simulink model "DC_Microgrid_Sim"  (R2023b)
settings: Solver=VariableStepDiscrete  StartTime=0.0  StopTime=720  MaxStep=1e2  RelTol=1e-3
undefined symbols (not defined in the file or in its folder): Ion, Lithium, Ts_Control, Ts_Power
libraries: spsSeriesRLCBranchLib x5, spsVoltageMeasurementLib x3, spsCurrentMeasurementLib x2, spsMosfetLib x2, SignalEditorBlockLib x2, spsDiodeLib x2, spsFirstOrderFilterLib x2, spsBatteryLib x1, simulink x1, slpidlib x1, spsPWMGeneratorDCDCLib x1, spsVariableResistorLib x1
settings Model: SimulationMode=accelerator  Creator=andrewboland  LastModifiedBy=andrewboland

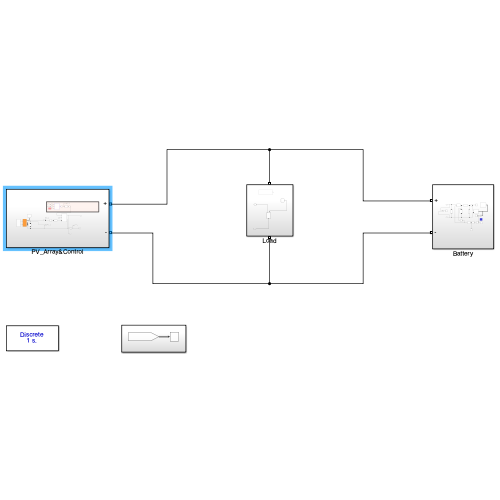
[thumbnail: Simulink's stored preview of the top-level diagram]
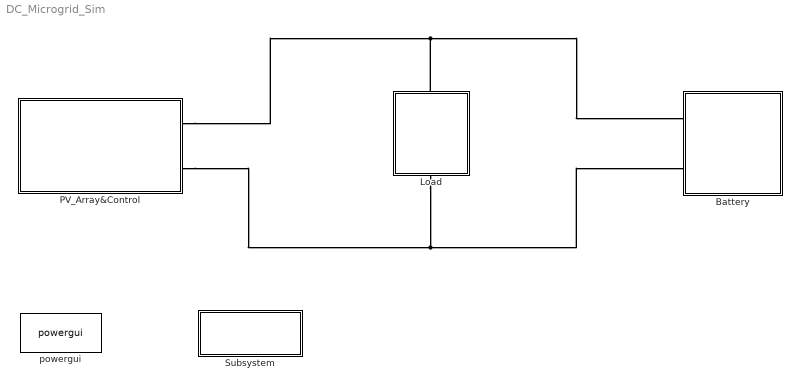
== system DC_Microgrid_Sim ==
  Battery : Subsystem
  Load : Subsystem
      settings: PortSchema="{\"entries\":[{\"content\":{\"sides\":[{\"content\":{},\"type\":\"ConnectorPlacement.EquallySpacedRectSide\",\"uuid\":\"223a8ec7-d9ac-4869-be30-0e3f111284b6\"},{\"content\":{\"side\":\"RIGHT\"},\"type\":\"ConnectorPlacement.EquallySpacedRectSide\",\"uuid\":\"4171ceb5-df16-4550-9af5-4849cdd8fb69\"},{\"content\":{\"connectorIds\":[\"LConn1\"],\"side\":\"TOP\"},\"type\":\"ConnectorPlacement.EquallySpacedRectSide\",\"uuid\":\"6a035cfa-8de8-4480-8689-7e250be4b844\"},{\"content\":{\"connectorIds\":[\"RConn1\"],\"side\":\"BOTTOM\"},\"type\":\"ConnectorPlacement.EquallySpacedRectSide\",\"uuid\":\"833ff93c-2ddd-4d5a-b476-72d44fccdab2\"}]},\"type\":\"ConnectorPlacement.EquallySpacedConnector\",\"uuid\":\"7d183c8c-61a7-4d89-b167-90b7ffe5dbe5\"}],\"packageUris\":[\"http://schema.mathworks.com/mf0/Connector/R2020b\"],\"version\":\"1.0\"}"
  PV_Array&Control : Subsystem
  Subsystem : Subsystem
  powergui : spspowerguiLib/powergui  Priority=1  SimulationMode=Discrete  SampleTime=1  frequency=60  Iterations=50  frequencyindice=0  Pbase=100e6  ErrMax=1e-4  UnitsV=kV  UnitsW=MW  buscounter=0  FunctionMessages=off  echomessages=off  EnableUseOfTLC=off  CurrentSourceSwitches=off  DisableSnubberDevices=off  DisableRonSwitches=off  DisableVfSwitches=off  DisplayEquations=off  AutomaticDiscreteSolvers=off  SolverType=Tustin/Backward Euler (TBE)  Interpol=off  ExternalGateDelay=off  methode=off  Ts=100  x0status=blocks  SPID=on  SwTol=0  HookPort=off  NonlinearTolerance=1e-4  nMaxIteration=100  ContinueOnMaxIteration=off  RestoreLinks=warning  ResistiveCurrentMeasurement=off  Frange=[0:2:500]  Ylog=off  Xlog=on  ShowGrid=off  save=off  variable=ZData  structure=0  ZoomFFT=off  StartTime=0.0  cycles=1  DisplayStyle=1  fundamental=60  FreqAxis=off  MaxFrequency=1000  frequencyindicesteady=1  RmsSteady=1  display=off
  connections:
  PV_Array&Control/RConn1 -- Load/LConn1 -- Battery/LConn1
  PV_Array&Control/RConn2 -- Load/RConn1 -- Battery/LConn2

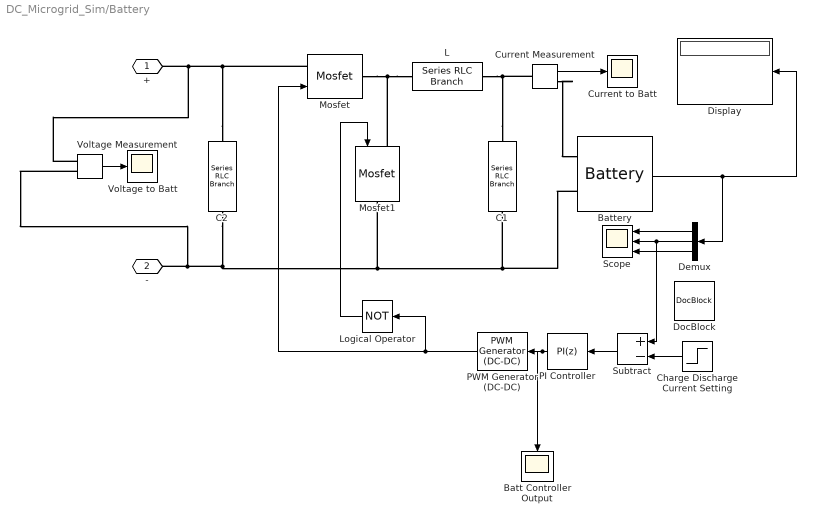
== system DC_Microgrid_Sim/Battery ==
  Batt Controller Output : Scope
  Battery : spsBatteryLib/Battery  BatType=Lithium-Ion  ShowTempParam=off  ThermalPreset=no  ShowAgeParam=off  NomV=400  NomQ=360  SOC=50  Batt_Tr=1  PresetModel=on  MaxQ=360  MinV=300  FullV=465.5949  Dis_rate=156.5217  R=0.011111  Normal_OP=325.5652  expZone="[432.1543      17.68696]"  current=[6.5 13 32.5]  Units=Time  Tci=20  NomT=25  T2=0  MaxQ2=2.208  FullV2=3.45  Normal_OP2=2.8  expZone2="[3.22        0.23]"  Rca=0.6  ti=1000  Dp=0  Neq0=0  Tsim=1e6  Ta1=25  Qeol=5.4*0.9  Reol=0.013333*1.2  Char_age=[2.3478, 3]  Dis_age=[2.3478, 10]  N1=1500  N2=10500  N3=1000  N4=1400  Ta2=45  N5=950
      settings: LibrarySourceBlock=electricdrivelib/Extra Sources/Battery
  C1 : spsSeriesRLCBranchLib/Series RLC Branch  LConnTagsString=__new0  RConnTagsString=__new0  BranchType=RC  Resistance=1e-3  Inductance=1e-3  SetiL0=off  InitialCurrent=0  Capacitance=1000e-6  Setx0=off  InitialVoltage=0  Measurements=None
  C2 : spsSeriesRLCBranchLib/Series RLC Branch  LConnTagsString=__new0  RConnTagsString=__new0  BranchType=RC  Resistance=1e-3  Inductance=1e-3  SetiL0=off  InitialCurrent=0  Capacitance=1000e-6  Setx0=off  InitialVoltage=0  Measurements=None
  Charge Discharge Current Setting : Step  Before=5  After=-5  SampleTime=0
  Current Measurement : spsCurrentMeasurementLib/Current Measurement  PhasorSimulation=off  OutputType=Complex  PSBequivalent=0
  Current to Batt : Scope
  Demux : Demux  Outputs=3
  Display : Display
  DocBlock : simulink/Model-Wide Utilities/DocBlock  DocumentType=Text
      content=|
      | Half Bridge Bidirectional DC-DC Converter with PI Current Control Demo
      | Developed by Rodney Tan (PhD)
      | Version 1.00 (July 2019)
      |
      | This Simulink model demonstrate a non-isolated half bridge Bidirectional
      | DC-DC Converter with PI current control typically used for battery charge
      | discharge control application.
      |
      | The charge and discharge mode is control by the charge discharge current
      | setting block where a positive current set the converter to discharging mode
      | and a negative current set the converter to charging mode.
  L : spsSeriesRLCBranchLib/Series RLC Branch  LConnTagsString=__new0  RConnTagsString=__new0  BranchType=L  Resistance=0.1  Inductance=100e-6  SetiL0=off  InitialCurrent=0  Capacitance=1e-6  Setx0=off  InitialVoltage=0  Measurements=None
  Logical Operator : Logic  Operator=NOT  AllPortsSameDT=off  OutDataTypeStr=boolean
  Mosfet : spsMosfetLib/Mosfet  Ron=0.1  Lon=0  Rd=0.01  Vfd=0  IC=0  Rs=1e5  Cs=inf  Measurements=off
  Mosfet1 : spsMosfetLib/Mosfet  Ron=0.1  Lon=0  Rd=0.01  Vfd=0  IC=0  Rs=1e5  Cs=inf  Measurements=off
  PI Controller : slpidlib/PID Controller  Controller=PI  Form=Parallel  TimeDomain=Discrete-time  UseExternalTs=off  SampleTime=-1  IntegratorMethod=Forward Euler  FilterMethod=Forward Euler  ControllerParametersSource=internal  P=0.01  I=5  UseKiTs=off  D=0  N=0  UseFilter=on  TunerSelectOption=Transfer Function Based (PID Tuner App)  InitialConditionSource=internal  InitialConditionForIntegrator=0  InitialConditionForFilter=0  DifferentiatorICPrevScaledInput=0  ExternalReset=none  TrackingMode=off  Kt=1  LimitOutput=on  SatLimitsSource=internal  UpperSaturationLimit=0.9  LowerSaturationLimit=0  LinearizeAsGain=on  AntiWindupMode=none  Kb=1  LimitIntegrator=off  UpperIntegratorSaturationLimit=inf  LowerIntegratorSaturationLimit=-inf  POutMin=[]  POutMax=[]  IOutMin=[]  IOutMax=[]  DOutMin=[]  DOutMax=[]  NOutMin=[]  NOutMax=[]  SumOutMin=[]  SumOutMax=[]  SaturationOutMin=[]  SaturationOutMax=[]  PParamMin=[]  PParamMax=[]  IParamMin=[]  IParamMax=[]  DParamMin=[]  DParamMax=[]  NParamMin=[]  NParamMax=[]  KbParamMin=[]  KbParamMax=[]  KtParamMin=[]  KtParamMax=[]  KbOutMin=[]  KbOutMax=[]  KtOutMin=[]  KtOutMax=[]  IntegratorOutMin=[]  IntegratorOutMax=[]  FilterOutMin=[]  FilterOutMax=[]  SumI1OutMin=[]  SumI1OutMax=[]  SumI2OutMin=[]  SumI2OutMax=[]  SumI3OutMin=[]  SumI3OutMax=[]  SumI4OutMin=[]  SumI4OutMax=[]  SumDOutMin=[]  SumDOutMax=[]  DifferentiatorOutMin=[]  DifferentiatorOutMax=[]  FilterDiffOutCoefMin=[]  FilterDiffOutCoefMax=[]  ReciprocalOutMin=[]  ReciprocalOutMax=[]  SumDenOutMin=[]  SumDenOutMax=[]  SumNumOutMin=[]  SumNumOutMax=[]  DivideOutMin=[]  DivideOutMax=[]  UdiffTsProdOutMin=[]  UdiffTsProdOutMax=[]  NTsProdOutMin=[]  NTsProdOutMax=[]  UintegralTsProdOutMin=[]  UintegralTsProdOutMax=[]  UngainTsProdOutMin=[]  UngainTsProdOutMax=[]  ClampingZeroOutDataTypeStr=Inherit: Inherit via back propagation  ClampingZeroOutMin=[]  ClampingZeroOutMax=[]  FilterDenConstantOutDataTypeStr=Inherit: Inherit via back propagation  FilterDenConstantOutMin=[]  FilterDenConstantOutMax=[]  PCopyOutDataTypeStr=Inherit: Inherit via back propagation  PCopyOutMin=[]  PCopyOutMax=[]  NCopyOutDataTypeStr=Inherit: Inherit via back propagation  NCopyOutMin=[]  NCopyOutMax=[]  IntegratorContinuousStateAttributes=''  IntegratorStateMustResolveToSignalObject=off  IntegratorRTWStateStorageClass=Auto  FilterContinuousStateAttributes=''  FilterStateMustResolveToSignalObject=off  FilterRTWStateStorageClass=Auto  ParallelPVariant=InternalParameters  IdealPVariant=Disabled  IVariant=InternalParameters  DVariant=Disabled  IntegratorVariant=Discrete  SatVariant=Enabled  AWVariant=Passthrough  PCopyVariant=Disabled  TRVariant=Disabled  FdbkBlocksVariant=Forward  IdealPFdbkVariant=Disabled  SatFdbkVariant=Disabled  DerivativeFilterVariant=Disabled  NVariant=Disabled  NCopyVariant=Disabled_SignalSpec  FilterICVariant=Disabled  IntegratorICVariant=InternalICs  ExternalResetVariant=Disabled  TRSumVariant=Passthrough  SumFdbkVariant=Disabled  SumVariant=Sum_PI  TsampFilterVariant=InternalTs  TsampNgainVariant=Passthrough  TsampIntegralVariant=Disabled_SignalSpec  ExternalSaturationOutDataTypeStr=Inherit: Same as second input
  PWM Generator (DC-DC) : spsPWMGeneratorDCDCLib/PWM Generator (DC-DC)  Fsw=10e3  Ts=0
  Scope : Scope  NumInputPorts=3
  Subtract : Sum  Inputs=+-
  Voltage Measurement : spsVoltageMeasurementLib/Voltage Measurement  PhasorSimulation=off  OutputType=Complex  PSBequivalent=0
  Voltage to Batt : Scope
  + : PMIOPort  Side=Left
  - : PMIOPort  Port=2  Side=Left
  wires:
  Demux/3 -> Scope/3
  Demux/2 -> Subtract/1, Scope/2
  Demux/1 -> Scope/1
  Subtract/1 -> PI Controller/1
  Logical Operator/1 -> Mosfet1/1
  PI Controller/1 -> Batt Controller Output/1, PWM Generator (DC-DC)/1
  Charge Discharge Current Setting/1 -> Subtract/2
  Battery/1 -> Display/1, Demux/1
  PWM Generator (DC-DC)/1 -> Mosfet/1, Logical Operator/1
  Voltage Measurement/1 -> Voltage to Batt/1
  Current Measurement/1 -> Current to Batt/1
  connections:
  C2/RConn1 -- Battery/LConn2 -- C1/RConn1 -- Mosfet1/RConn1 -- Voltage Measurement/LConn2 -- -/RConn1
  C2/LConn1 -- Voltage Measurement/LConn1 -- +/RConn1 -- Mosfet/LConn1
  L/LConn1 -- Mosfet/RConn1 -- Mosfet1/LConn1
  C1/LConn1 -- Current Measurement/LConn1 -- L/RConn1
  Current Measurement/RConn1 -- Battery/LConn1

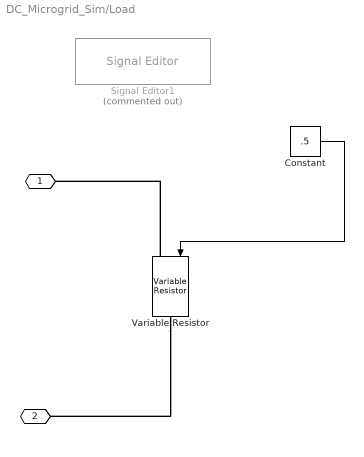
== system DC_Microgrid_Sim/Load ==
  Constant : Constant  Value=.5
  Signal Editor1 : SignalEditorBlockLib/Signal Editor  Commented=on  FileName=load_signal.mat  ActiveScenario=scenario  ActiveSignal=Resistance  IsBus=off  OutputBusObjectStr=Bus: BusObject  SampleTime=0  Interpolate=off  ZeroCross=off  OutputAfterFinalValue=Setting to zero  Unit=inherit  PreserveSignalName=on  ApplySigPropsToAllScenarios=on  ApplySigPropsToAllSignals=off
  Variable Resistor : spsVariableResistorLib/Variable Resistor  Rabsmin=1e-3
      settings: LibrarySourceBlock=sps_lib/Passives/Variable Resistor
  " " : PMIOPort  Side=Left
  "  " : PMIOPort  Port=2  Side=Right
  wires:
  Constant/1 -> Variable Resistor/1
  connections:
  Variable Resistor/RConn1 -- "  "/RConn1
  Variable Resistor/LConn1 -- " "/RConn1

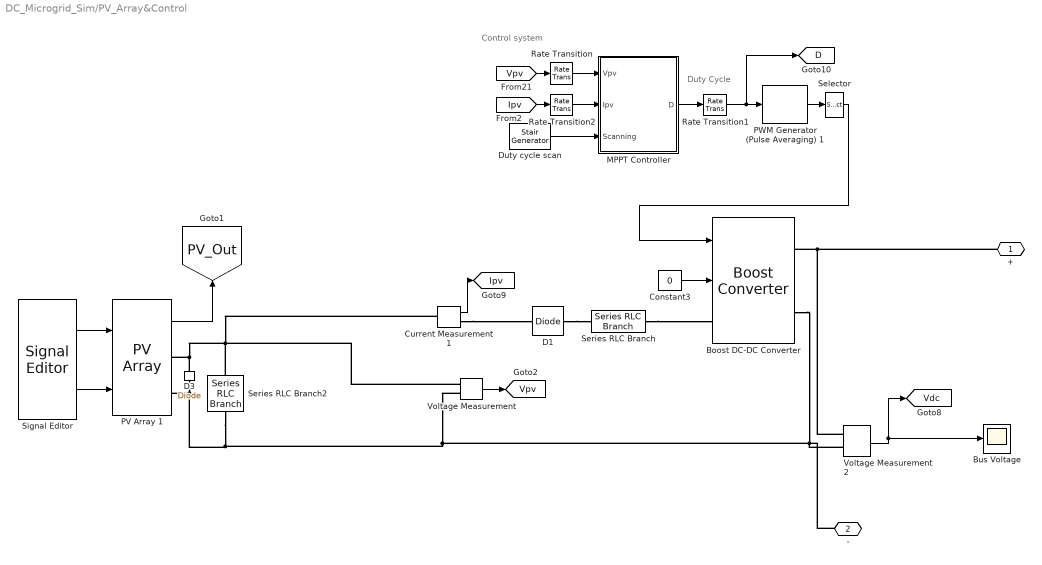
== system DC_Microgrid_Sim/PV_Array&Control ==
  note: Control system
  note: Duty Cycle
  Boost DC-DC Converter : spsBoostConverterLib/Boost Converter  ModelType=Switching function  Ron=1e-3  Rs=1e6  Cs=inf  Vforward=[0,0]  Ron_Diode=1e-3  Rs_Diode=1e6  Cs_Diode=inf  Vf_Diode=0  Rs_CurrentSource=inf  Ron_ACsource=1e-3
  Bus Voltage : Scope
  Constant3 : Constant  Value=0
  Current Measurement1 : spsCurrentMeasurementLib/Current Measurement  PhasorSimulation=off  OutputType=Complex  PSBequivalent=0
  D1 : spsDiodeLib/Diode  Ron=1e-3  Lon=0  Vf=Vf_Diode  IC=0  UseSnubber=0  Rs=1e6  Cs=inf  Measurements=off
  D3 : spsDiodeLib/Diode  Ron=1e-3  Lon=0  Vf=.6  IC=0  UseSnubber=0  Rs=1e6  Cs=inf  Measurements=off
  Duty cycle scan : spsStairGeneratorLib/Stair Generator  t=[0,0.40, 0.41]  e=[0, 1, 0]  Ts=Ts_Control
  MPPT Controller : Subsystem  mask(MPPT Controller - Perturb and Observe algorithm (PandO)){Dinit=0.39, Dlimits=[0.85, 0.30], deltaD=50e-6, Fc=1000, ScanDuration=0.25, Ts=Ts_Control}
      mask prompts: Dinit "Duty cycle (D) initial value"; Dlimits "D limits [Upper, Lower]"; deltaD "Increment value for PandO algorithm"; Fc "Measurement filter cutoff frequency (Hz)"; ScanDuration "Scanning mode duration (s)"; Ts "Sample time (s)"
      mask init:
      | Dmax=Dlimits(1);
      | Dmin=Dlimits(2);
      | SampleTime=Ts;
      | DeltaD_Scan=(Dmax-Dmin)*Ts/ScanDuration;
  PV Array 1 : spsPVArrayLib/PV Array  Npar=64  Nser=4  PlotType=array @ 1000 W/m2 & specified temperatures  S_vec="[ 1000  500  100 ]"  Temp_C_vec="[ 45 25  ]"  ModuleName=SunPower SPR-315E-WHT-D  PlotWhenSelected=off  Pm=315.072  Ncell=96  Voc=64.6  Isc=6.14  Vm=54.7  Im=5.76  beta_Voc_pc=-0.2727  alpha_Isc_pc=0.061743  beta_Voc=-0.17616  alpha_Isc=0.003791  IL=6.1461  I0=6.5067e-12  nI=0.95071  Rsh=430.0666  Rs=0.43041  RobustModel=off  RobustCellTemperature=40  BAL=on  Tc=1e-6  Tfilter=5e-5
  PWM Generator (Pulse Averaging) 1 : spsPWMGeneratorPulseAveragingLib/PWM Generator (Pulse Averaging)  GeneratorType=Two-quadrant  Fc=20e3  InitialPhase=90  Ts=Ts_Power
  Rate Transition : RateTransition  OutPortSampleTime=Ts_Control
  Rate Transition1 : RateTransition  OutPortSampleTime=Ts_Power
  Rate Transition2 : RateTransition  OutPortSampleTime=Ts_Control
  Selector : Selector  InputPortWidth=2  IndexOptions=Index vector (dialog)  Indices=1  OutputSizes=1
  Series RLC Branch : spsSeriesRLCBranchLib/Series RLC Branch  LConnTagsString=__new0  RConnTagsString=__new0  BranchType=RL  Resistance=20e-3  Inductance=20e-3  SetiL0=off  InitialCurrent=0  Capacitance=1e-6  Setx0=off  InitialVoltage=0  Measurements=None
  Series RLC Branch2 : spsSeriesRLCBranchLib/Series RLC Branch  LConnTagsString=__new0  RConnTagsString=__new0  BranchType=C  Resistance=10e-3  Inductance=10e-3  SetiL0=off  InitialCurrent=0  Capacitance=10e-6  Setx0=off  InitialVoltage=0  Measurements=None
  Signal Editor : SignalEditorBlockLib/Signal Editor  FileName=pv_signals.mat  ActiveScenario=scenario  ActiveSignal=Irradiance  IsBus=off  OutputBusObjectStr=Bus: BusObject  SampleTime=0  Interpolate=off  ZeroCross=off  OutputAfterFinalValue=Setting to zero  Unit=inherit  PreserveSignalName=on  ApplySigPropsToAllScenarios=on  ApplySigPropsToAllSignals=off
  Voltage Measurement : spsVoltageMeasurementLib/Voltage Measurement  PhasorSimulation=off  OutputType=Complex  PSBequivalent=0
  Voltage Measurement2 : spsVoltageMeasurementLib/Voltage Measurement  PhasorSimulation=off  OutputType=Complex  PSBequivalent=0
  + : PMIOPort  Side=Right
  - : PMIOPort  Port=2  Side=Right
  tag scope: D=global, Ipv=global, PV_Out=global, Vdc=global, Vpv=global
  wires:
  Signal Editor/1 -> PV Array 1/1
  PV Array 1/1 -> [PV_Out]
  Signal Editor/2 -> PV Array 1/2
  Voltage Measurement/1 -> [Vpv]
  Rate Transition/1 -> MPPT Controller/1(Vpv)
  [Ipv] -> Rate Transition2/1
  Duty cycle scan/1 -> MPPT Controller/3(Scanning)
  Rate Transition1/1 -> [D], PWM Generator (Pulse Averaging) 1/1
  MPPT Controller/1(D) -> Rate Transition1/1
  Current Measurement1/1 -> [Ipv]
  Rate Transition2/1 -> MPPT Controller/2(Ipv)
  Selector/1 -> Boost DC-DC Converter/1
  PWM Generator (Pulse Averaging) 1/1 -> Selector/1
  [Vpv] -> Rate Transition/1
  Constant3/1 -> Boost DC-DC Converter/2
  Voltage Measurement2/1 -> Bus Voltage/1, [Vdc]
  connections:
  Series RLC Branch2/LConn1 -- Voltage Measurement/LConn1 -- Current Measurement1/LConn1 -- D3/RConn1 -- PV Array 1/RConn1
  Voltage Measurement/LConn2 -- -/RConn1 -- Voltage Measurement2/LConn2 -- Boost DC-DC Converter/RConn2 -- D3/LConn1 -- PV Array 1/RConn2 -- Series RLC Branch2/RConn1
  Voltage Measurement2/LConn1 -- +/RConn1 -- Boost DC-DC Converter/RConn1
  D1/RConn1 -- Series RLC Branch/LConn1
  Series RLC Branch/RConn1 -- Boost DC-DC Converter/LConn1
  Current Measurement1/RConn1 -- D1/LConn1

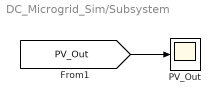
== system DC_Microgrid_Sim/Subsystem ==
  PV_Out : Scope
  wires:
  [PV_Out] -> PV_Out/1

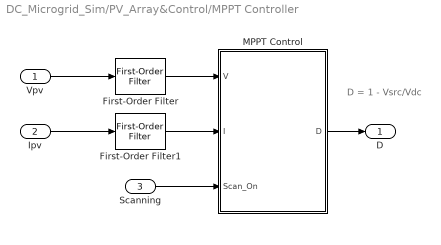
== system DC_Microgrid_Sim/PV_Array&Control/MPPT Controller ==
  note: D = 1 - Vsrc/Vdc
  Vpv : Inport
  Ipv : Inport  Port=2
  Scanning : Inport  Port=3  PortDimensions=1
  First-Order Filter : spsFirstOrderFilterLib/First-Order Filter  FilterType=Lowpass  Tc=1/Fc  Ts=Ts  Initialize=off  Vac_Init=[0, 0, 60]  Vdc_Init=0  PlotResponse=off  FreqRange="[0,  200,  1]"
  First-Order Filter1 : spsFirstOrderFilterLib/First-Order Filter  FilterType=Lowpass  Tc=1/Fc  Ts=Ts  Initialize=off  Vac_Init=[0, 0, 60]  Vdc_Init=0  PlotResponse=off  FreqRange="[0,  200,  1]"
  MPPT Control : MATLAB Function  TreatAsAtomicUnit=on
  D : Outport  OutDataTypeStr=double  PortDimensions=1  VectorParamsAs1DForOutWhenUnconnected=off
  wires:
  First-Order Filter1/1 -> MPPT Control/2(I)
  First-Order Filter/1 -> MPPT Control/1(V)
  Ipv/1 -> First-Order Filter1/1
  Vpv/1 -> First-Order Filter/1
  MPPT Control/1(D) -> D/1
  Scanning/1 -> MPPT Control/3(Scan_On)

== matlab function DC_Microgrid_Sim/PV_Array&Control/MPPT Controller/MPPT Control ==
  settings: updateMethod=DISCRETE  sampleTime=Ts
  data: V input =V; I input; D output; Dmax parameter; Dmin parameter; deltaD parameter; Dinit parameter; Scan_On input; DeltaD_Scan parameter
function D   = PandO(V, I, Dmax, Dmin, deltaD, Dinit, Scan_On, DeltaD_Scan)

% MPPT controller based on the Perturb & Observe algorithm.

% D output = Duty cycle of the boost converter (value between 0 and 1)
% V input = PV array terminal voltage (V)
% I input = PV array current (A)
% D = 1 - Vinput/Voutput (increasing D decrease Vin)

persistent Vold Pold Dold Scan_On_Old Pmax D_Pmax V_Pmax;
%
if isempty(Vold)
    Vold=0;
    Pold=0;
    Scan_On_Old=0;
    Dold=Dinit;
    Pmax=0;
    D_Pmax=0;
    V_Pmax=0;
end
P= V*I;
if Scan_On==1 || Scan_On_Old==1
    if Scan_On_Old==0
        Scan_On_Old=1;
        D=Dmin;
    else
        D=Dold+DeltaD_Scan;
    end
    Dold=D;
    if P>Pmax
        Pmax=P;
        D_Pmax=D;
    end
    if D >= Dmax
        Scan_On_Old=0;
        Pold=Pmax;
        Dold=D_Pmax;
        Vold=V_Pmax;
    end
else
    dV= V - Vold;
    dP= P - Pold;
    %
    if dP ~= 0
        if dP < 0
            if dV < 0
                D = Dold - deltaD;
            else
                D = Dold + deltaD;
            end
        else
            if dV < 0
                D = Dold + deltaD;
            else
                D = Dold - deltaD;
            end
        end
    else
        D=Dold;
    end
    %
    if D >= Dmax || D<= Dmin
        D=Dold;
    end
    %
    Dold=D;
    Vold=V;
    Pold=P;
end
